simulink model "LinearTopTest"  (R2019a)
settings: Solver=FixedStepAuto  StartTime=0.0  StopTime=10  FixedStep=h  RelTol=1e-3
values from neighbouring files (symbols this model uses):
  firstLocation = [0 0]    [testingLQRDisturbance.m]    (also in testingObserver.m = [ 0 0]; testingPoleController.m = [ -0.3 0.3]; testingPoleControllerDisturbance.m; testingreftrackingLQR.m)
  Parameters = CoenParams(X)    [EstimatedParams.m]    (also in LQR.m = EstimatedParams(); LSQnonLinfunc.m; TestModel.m = CoenParams(X0); testingLQRDisturbance.m = EstimatedParams())
settings Model: Creator=coeng  LastModifiedBy=coeng
settings DebuggingCC: ArithmeticOperatorsInVariantConditions=warning
settings CodeAppCC: StateflowObjectComments=on

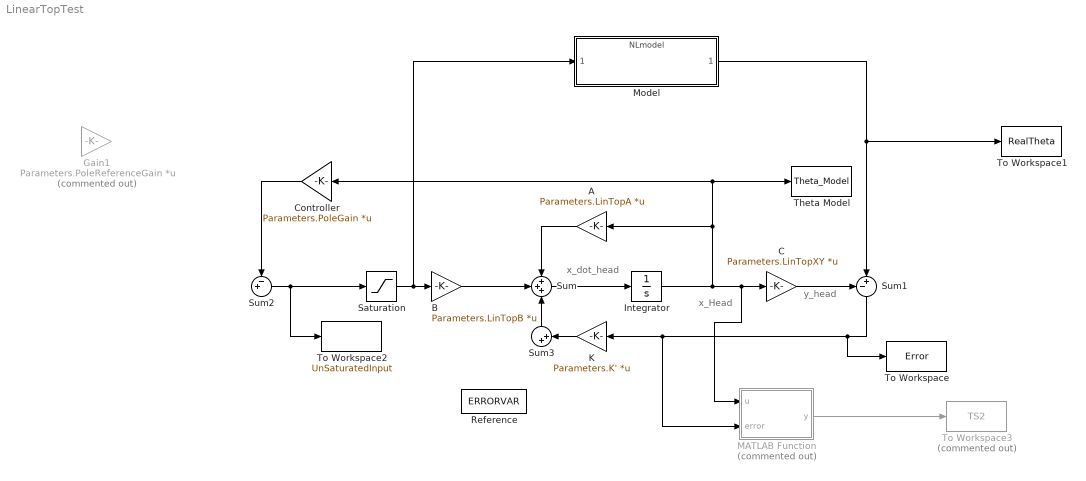
== system LinearTopTest ==
  note: y_head
  note: x_dot_head
  note: x_Head
  A : Gain  Gain=Parameters.LinTopA  Multiplication=Matrix(K*u)
  B : Gain  Gain=Parameters.LinTopB  Multiplication=Matrix(K*u)
  C : Gain  Gain=Parameters.LinTopXY  Multiplication=Matrix(K*u)
  Controller : Gain  Gain=Parameters.PoleGain  Multiplication=Matrix(K*u)
  Gain1 : Gain  Commented=on  Gain=Parameters.PoleReferenceGain  Multiplication=Matrix(K*u)
  Integrator : Integrator  InitialCondition=[0; firstLocation'; 0; 0]
  K : Gain  Gain=Parameters.K'  Multiplication=Matrix(K*u)
  MATLAB Function : MATLAB Function  Commented=on  TreatAsAtomicUnit=on
  Model : ModelReference  ModelNameDialog=NLmodel  SimulationMode=Normal  ModelReferenceVersion=1.67
  "Reference " : FromWorkspace  VariableName=ERRORVAR  SampleTime=0
  Saturation : Saturate  UpperLimit=1  LowerLimit=-1
  Sum : Sum  Inputs=+++
  Sum1 : Sum  Inputs=-+|
  Sum2 : Sum  Inputs=-+|
  Sum3 : Sum  Inputs=|++
  Theta Model : ToWorkspace  VariableName=Theta_Model  SaveFormat=Timeseries  SampleTime=-1
  To Workspace : ToWorkspace  VariableName=Error  SaveFormat=Timeseries  SampleTime=-1
  To Workspace1 : ToWorkspace  VariableName=RealTheta  SaveFormat=Timeseries  SampleTime=-1
  To Workspace2 : ToWorkspace  VariableName=UnSaturatedInput  SaveFormat=Timeseries  SampleTime=-1
  To Workspace3 : ToWorkspace  Commented=on  VariableName=TS2  SaveFormat=Timeseries  SampleTime=-1
  wires:
  Sum/1 -> Integrator/1
  Integrator/1 -> MATLAB Function/1(u), C/1, A/1, Controller/1, Theta Model/1
  Sum2/1 -> To Workspace2/1, Saturation/1
  Saturation/1 -> Model/1, B/1
  Sum1/1 -> MATLAB Function/2(error), K/1, To Workspace/1
  C/1 -> Sum1/1
  Controller/1 -> Sum2/1
  A/1 -> Sum/1
  B/1 -> Sum/2
  Model/1 -> Sum1/2, To Workspace1/1
  K/1 -> Sum3/2
  Sum3/1 -> Sum/3
  MATLAB Function/1(y) -> To Workspace3/1

== matlab function LinearTopTest/MATLAB Function ==
  data: u input; y output; error input
function y = fcn(u, error)
err2 = error
y = u
